simulink model "bloques"  (R2021b)
settings: Solver=FixedStepAuto  StartTime=0.0  StopTime=Tc  FixedStep=Ts  RelTol=1e-3
values from neighbouring files (symbols this model uses):
  a = 12.650058*Ts*Ts    (= 1.2650058e-07)    [raiz.m]
  b = 20.8968*Ts - 2    (= -1.99791032)    [raiz.m]
  c = 1 - 20.8968*Ts    (= 0.99791032)    [raiz.m]
  Kp = 16.6742    [raiz.m]
  sp = 100    [raiz.m]
  Tz = 0.001    [raiz.m]
settings Model: Creator=yeezvs  LastModifiedBy=yeezvs
settings DataIOCC: ReturnWorkspaceOutputs=off

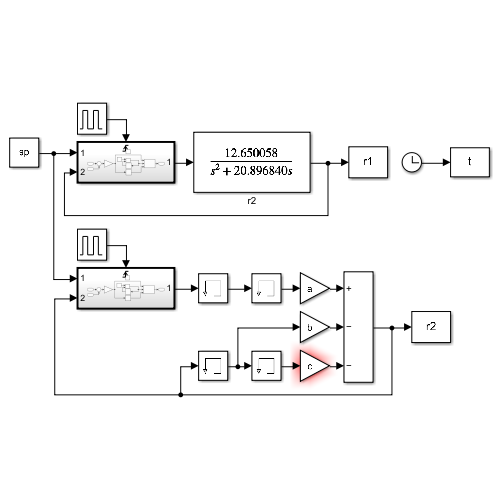
[thumbnail: Simulink's stored preview of the top-level diagram]
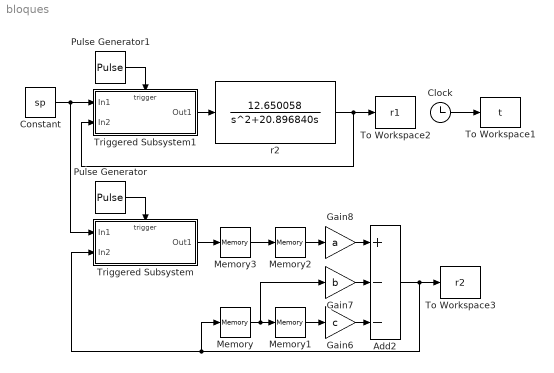
== system bloques ==
  Add2 : Sum  Inputs=+|-|-
  Clock : Clock
  Constant : Constant  Value=sp
  Gain6 : Gain  Gain=c
  Gain7 : Gain  Gain=b
  Gain8 : Gain  Gain=a
  Memory{,1..3} (4 alike) : Memory
  Pulse Generator : DiscretePulseGenerator  PulseType=Time based  Period=Tz  PulseWidth=50
  Pulse Generator1 : DiscretePulseGenerator  PulseType=Time based  Period=Tz  PulseWidth=50
  To Workspace1 : ToWorkspace  VariableName=t  SampleTime=-1
  To Workspace2 : ToWorkspace  VariableName=r1  SampleTime=-1
  To Workspace3 : ToWorkspace  VariableName=r2  SampleTime=-1
  Triggered Subsystem : Subsystem  TreatAsAtomicUnit=on
  Triggered Subsystem1 : Subsystem  TreatAsAtomicUnit=on
  r2 : TransferFcn  Numerator=[12.650058]  Denominator=[1 20.896840 0]
  wires:
  Clock/1 -> To Workspace1/1
  Triggered Subsystem1/1(Out1) -> r2/1
  Gain8/1 -> Add2/1
  Constant/1 -> Triggered Subsystem/1(In1), Triggered Subsystem1/1(In1)
  Add2/1 -> To Workspace3/1, Triggered Subsystem/2(In2), Memory/1
  r2/1 -> Triggered Subsystem1/2(In2), To Workspace2/1
  Pulse Generator/1 -> Triggered Subsystem/Trigger
  Pulse Generator1/1 -> Triggered Subsystem1/Trigger
  Memory2/1 -> Gain8/1
  Memory3/1 -> Memory2/1
  Triggered Subsystem/1(Out1) -> Memory3/1
  Gain7/1 -> Add2/2
  Gain6/1 -> Add2/3
  Memory1/1 -> Gain6/1
  Memory/1 -> Gain7/1, Memory1/1

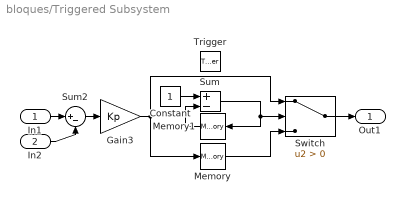
== system bloques/Triggered Subsystem ==
  In1 : Inport
  In2 : Inport  Port=2
  Trigger : TriggerPort  VariantControl=(inherit)
  Constant : Constant
  Gain3 : Gain  Gain=Kp
  Memory : Memory  InheritSampleTime=on
  Memory1 : Memory  InheritSampleTime=on
  Sum : Sum  Inputs=+-  InputSameDT=on  SaturateOnIntegerOverflow=on  OutDataTypeStr=Inherit: Same as first input
  Sum2 : Sum  Inputs=|+-
  Switch : Switch  Criteria=u2 > Threshold
  Out1 : Outport
  wires:
  Sum2/1 -> Gain3/1
  In1/1 -> Sum2/1
  In2/1 -> Sum2/2
  Gain3/1 -> Memory/1, Switch/1
  Memory/1 -> Switch/3
  Switch/1 -> Out1/1
  Sum/1 -> Memory1/1, Switch/2
  Memory1/1 -> Sum/2
  Constant/1 -> Sum/1

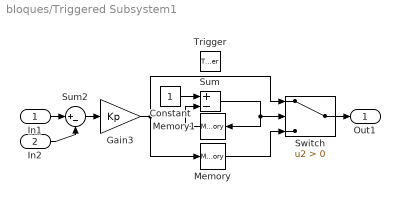
== system bloques/Triggered Subsystem1 ==
  In1 : Inport
  In2 : Inport  Port=2
  Trigger : TriggerPort  VariantControl=(inherit)
  Constant : Constant
  Gain3 : Gain  Gain=Kp
  Memory : Memory  InheritSampleTime=on
  Memory1 : Memory  InheritSampleTime=on
  Sum : Sum  Inputs=+-  InputSameDT=on  SaturateOnIntegerOverflow=on  OutDataTypeStr=Inherit: Same as first input
  Sum2 : Sum  Inputs=|+-
  Switch : Switch  Criteria=u2 > Threshold
  Out1 : Outport
  wires:
  Sum2/1 -> Gain3/1
  In1/1 -> Sum2/1
  In2/1 -> Sum2/2
  Gain3/1 -> Memory/1, Switch/1
  Memory/1 -> Switch/3
  Switch/1 -> Out1/1
  Sum/1 -> Memory1/1, Switch/2
  Memory1/1 -> Sum/2
  Constant/1 -> Sum/1
